simulink library "halout"  (R2021b)
settings: Solver=VariableStepAuto  StartTime=0.0  StopTime=10.0  RelTol=1e-3
undefined symbols (not defined in the file): C_TASK_5MS_S, FALSE, KHAL_CAN1FDAPS3E2E_flg, KHAL_CAN1FDAPS3TxReq_flg, KHAL_CAN1FDVCU2E2E_flg, KHAL_CAN1FDVCU2TxReq_flg, KHAL_CAN1FDVCU3E2E_flg, KHAL_CAN1FDVCU3TxReq_flg, KHAL_CAN1TxReq_flg, KHAL_CAN2TxReq_flg, KHAL_CAN3FDVCU1TxReq_flg, KHAL_CAN3FDVCU2E2E_flg, KHAL_CAN3FDVCU2TxReq_flg, KHAL_CAN3TxReq_flg, KHAL_CAN4FDVCU1E2E_flg, KHAL_CAN4FDVCU1TxReq_flg, KHAL_CAN4TxReq_flg, KHAL_CAN5TxReq_flg, ONE_INT, TRUE, ZERO_INT
libraries: FVT_lib x383, simulink x179
(part 2 of 20)

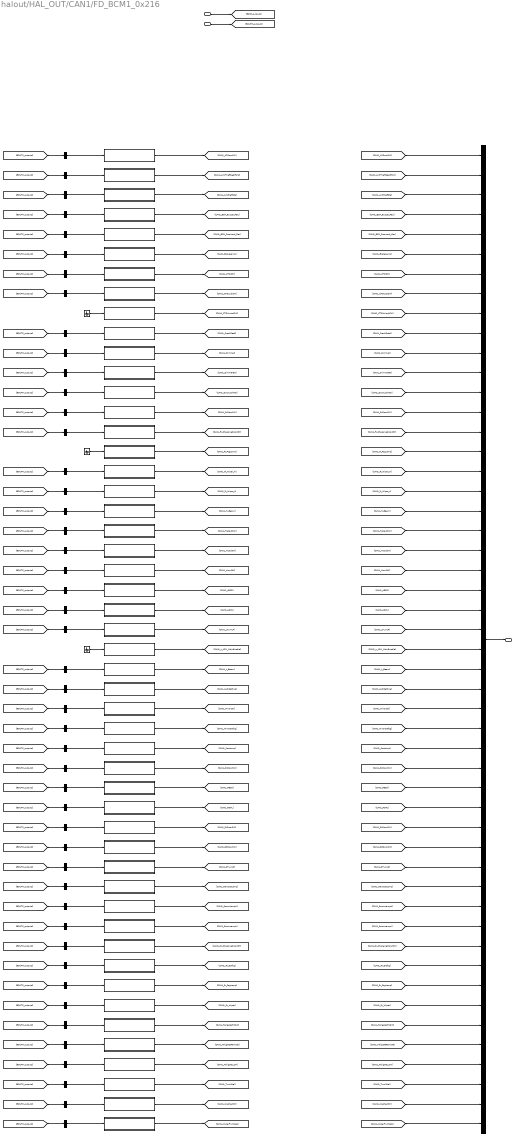
== system halout/HAL_OUT/CAN1/FD_BCM1_0x216 ==
  BSCP_outputs : Inport  OutDataTypeStr=Bus: BSCP_outputs
  BOUTP_outputs : Inport  Port=2  OutDataTypeStr=Bus: BOUTP_outputs
  AllDoorSW : Subsystem
  AntiTheftSeatFold : Subsystem
  AntitheftSta : Subsystem
  BCMBuzzerReq : Subsystem
  BCMDoorLockSta : Subsystem
  BrakeLamp : Subsystem
  CTDCtrl : Subsystem
  CTDLockSW : Subsystem
  CTDUnlockSW : Subsystem
  CrashDetd : Subsystem
  Dimmer : Subsystem
  DimmerEN : Subsystem
  DoorLockIND : Subsystem
  DrDoorSW : Subsystem
  FrChargingDoorCtrl : Subsystem
  FrFogLamp : Subsystem
  FrWiperH : Subsystem
  FrWiperL : Subsystem
  Ground : Ground
  Ground1 : Ground
  Ground2 : Ground
  HBeam : Subsystem
  HazardSW : Subsystem
  HoodSW : Subsystem
  HornCtrl : Subsystem
  LAPMWdwEnable : Subsystem
  LBSD : Subsystem
  LBeam : Subsystem
  LDRL : Subsystem
  LTurnLP : Subsystem
  LockSetting : Subsystem
  MirrorCtrl : Subsystem
  MirrorDefog : Subsystem
  PosLamp : Subsystem
  PsDoorSW : Subsystem
  RBSD : Subsystem
  RDRL : Subsystem
  RLDoorSW : Subsystem
  RRDoorSW : Subsystem
  RTurnLP : Subsystem
  ReverseLamp : Subsystem
  RoomLampH : Subsystem
  RoomLampL : Subsystem
  RrChargingDoorCtrl : Subsystem
  RrDefog : Subsystem
  RrFogLamp : Subsystem
  RrWiper : Subsystem
  TailgateHDSW : Subsystem
  TailgateRemote : Subsystem
  TailgateSW : Subsystem
  TrunkRel : Subsystem
  WasherCtrl : Subsystem
  WiperFixMode : Subsystem
  bus_creator : BusCreator  Inputs=50  OutDataTypeStr=Bus: DT_CAN1_SG_FD_BCM1  NonVirtualBus=on
  bus_selector : BusSelector  OutputSignals=VOUTP_AllDoorSW_flg
  bus_selector1 : BusSelector  OutputSignals=VOUTP_AntitheftSeatFlod_flg
  bus_selector10 : BusSelector  OutputSignals=VOUTP_DimmerEN_flg
  bus_selector11 : BusSelector  OutputSignals=VOUTP_DoorLockIND_flg
  bus_selector12 : BusSelector  OutputSignals=VOUTP_DrDoorSW_flg
  bus_selector13 : BusSelector  OutputSignals=VOUTP_FrChargingDoorCtrl_enum
  bus_selector14 : BusSelector  OutputSignals=VOUTP_FrWiperH_flg
  bus_selector15 : BusSelector  OutputSignals=VOUTP_FrWiperL_flg
  bus_selector16 : BusSelector  OutputSignals=VOUTP_HBeam_flg
  bus_selector17 : BusSelector  OutputSignals=VOUTP_HazardSW_flg
  bus_selector18 : BusSelector  OutputSignals=VOUTP_HoodSW_flg
  bus_selector19 : BusSelector  OutputSignals=VOUTP_HornCtrl_flg
  bus_selector2 : BusSelector  OutputSignals=VOUTP_AntitheftSta_enum
  bus_selector20 : BusSelector  OutputSignals=VOUTP_LBSD_flg
  bus_selector21 : BusSelector  OutputSignals=VOUTP_LDRL_flg
  bus_selector22 : BusSelector  OutputSignals=VOUTP_LTurnLP_flg
  bus_selector23 : BusSelector  OutputSignals=VOUTP_LBeam_flg
  bus_selector24 : BusSelector  OutputSignals=VOUTP_LockSetting_flg
  bus_selector25 : BusSelector  OutputSignals=VOUTP_MirrorCtrl_enum
  bus_selector26 : BusSelector  OutputSignals=VOUTP_MirrorDefog_flg
  bus_selector27 : BusSelector  OutputSignals=VOUTP_PosLamp_flg
  bus_selector28 : BusSelector  OutputSignals=VOUTP_PsDoorSW_flg
  bus_selector29 : BusSelector  OutputSignals=VOUTP_RBSD_flg
  bus_selector3 : BusSelector  OutputSignals=VOUTP_BCMBuzzerReq_flg
  bus_selector30 : BusSelector  OutputSignals=VOUTP_RDRL_flg
  bus_selector31 : BusSelector  OutputSignals=VOUTP_RLDoorSW_flg
  bus_selector32 : BusSelector  OutputSignals=VOUTP_RRDoorSW_flg
  bus_selector33 : BusSelector  OutputSignals=VOUTP_RTurnLP_flg
  bus_selector34 : BusSelector  OutputSignals=VOUTP_ReverseLamp_flg
  bus_selector35 : BusSelector  OutputSignals=VOUTP_RoomLampH_flg
  bus_selector36 : BusSelector  OutputSignals=VOUTP_RoomLampL_flg
  bus_selector37 : BusSelector  OutputSignals=VOUTP_RrChargingDoorCtrl_enum
  bus_selector38 : BusSelector  OutputSignals=VOUTP_RrDefog_flg
  bus_selector39 : BusSelector  OutputSignals=VOUTP_RrFogLamp_flg
  bus_selector4 : BusSelector  OutputSignals=VOUTP_BCMDoorLockSta_flg
  bus_selector40 : BusSelector  OutputSignals=VOUTP_RrWiper_flg
  bus_selector41 : BusSelector  OutputSignals=VOUTP_TailgateHDSW_flg
  bus_selector42 : BusSelector  OutputSignals=VOUTP_TailgateRemote_enum
  bus_selector43 : BusSelector  OutputSignals=VOUTP_TailgateSW_flg
  bus_selector44 : BusSelector  OutputSignals=VOUTP_TrunkRel_flg
  bus_selector45 : BusSelector  OutputSignals=VOUTP_WasherCtrl_enum
  bus_selector46 : BusSelector  OutputSignals=VOUTP_WiperFixMode_flg
  bus_selector5 : BusSelector  OutputSignals=VOUTP_BrakeLamp_flg
  bus_selector6 : BusSelector  OutputSignals=VOUTP_CTDCtrl_enum
  bus_selector7 : BusSelector  OutputSignals=VOUTP_CTDLockSW_flg
  bus_selector8 : BusSelector  OutputSignals=VOUTP_CrashDetd_flg
  bus_selector9 : BusSelector  OutputSignals=VOUTP_Dimmer_pct
  FD_BCM1 : Outport
  wires:
  BSCP_outputs/1 -> [BSCP_outputs]
  BOUTP_outputs/1 -> [BOUTP_outputs]
  [CAN1_AllDoorSW] -> bus_creator/1  "CAN1_AllDoorSW"
  [CAN1_AntiTheftSeatFold] -> bus_creator/2  "CAN1_AntiTheftSeatFold"
  [CAN1_AntitheftSta] -> bus_creator/3  "CAN1_AntitheftSta"
  [CAN1_BCM_Buzzer_Req] -> bus_creator/4  "CAN1_BCM_Buzzer_Req"
  [CAN1_BCM_DoorLock_Sta] -> bus_creator/5  "CAN1_BCM_DoorLock_Sta"
  [CAN1_BrakeLamp] -> bus_creator/6  "CAN1_BrakeLamp"
  [CAN1_CTDCtrl] -> bus_creator/7  "CAN1_CTDCtrl"
  [CAN1_CTDLockSW] -> bus_creator/8  "CAN1_CTDLockSW"
  [CAN1_CTDUnlockSW] -> bus_creator/9  "CAN1_CTDUnlockSW"
  [CAN1_CrashDetd] -> bus_creator/10  "CAN1_CrashDetd"
  [CAN1_Dimmer] -> bus_creator/11  "CAN1_Dimmer"
  [CAN1_DimmerEN] -> bus_creator/12  "CAN1_DimmerEN"
  [CAN1_DoorLockIND] -> bus_creator/13  "CAN1_DoorLockIND"
  [CAN1_DrDoorSW] -> bus_creator/14  "CAN1_DrDoorSW"
  [CAN1_Fr_ChargingDoorCtrl] -> bus_creator/15  "CAN1_Fr_ChargingDoorCtrl"
  [CAN1_Fr_FogLamp] -> bus_creator/16  "CAN1_Fr_FogLamp"
  [CAN1_Fr_Wiper_H] -> bus_creator/17  "CAN1_Fr_Wiper_H"
  [CAN1_Fr_Wiper_L] -> bus_creator/18  "CAN1_Fr_Wiper_L"
  [CAN1_H_Beam] -> bus_creator/19  "CAN1_H_Beam"
  [CAN1_HazardSW] -> bus_creator/20  "CAN1_HazardSW"
  [CAN1_HoodSW] -> bus_creator/21  "CAN1_HoodSW"
  [CAN1_HornCtrl] -> bus_creator/22  "CAN1_HornCtrl"
  [CAN1_LBSD] -> bus_creator/23  "CAN1_LBSD"
  [CAN1_LDRL] -> bus_creator/24  "CAN1_LDRL"
  [CAN1_LTurnLP] -> bus_creator/25  "CAN1_LTurnLP"
  [CAN1_L_APM_WdwEnable] -> bus_creator/26  "CAN1_L_APM_WdwEnable"
  [CAN1_L_Beam] -> bus_creator/27  "CAN1_L_Beam"
  [CAN1_LockSetting] -> bus_creator/28  "CAN1_LockSetting"
  [CAN1_MirrorCtrl] -> bus_creator/29  "CAN1_MirrorCtrl"
  [CAN1_MirrorDefog] -> bus_creator/30  "CAN1_MirrorDefog"
  [CAN1_PosLamp] -> bus_creator/31  "CAN1_PosLamp"
  [CAN1_PsDoorSW] -> bus_creator/32  "CAN1_PsDoorSW"
  [CAN1_RBSD] -> bus_creator/33  "CAN1_RBSD"
  [CAN1_RDRL] -> bus_creator/34  "CAN1_RDRL"
  [CAN1_RLDoorSW] -> bus_creator/35  "CAN1_RLDoorSW"
  [CAN1_RRDoorSW] -> bus_creator/36  "CAN1_RRDoorSW"
  [CAN1_RTurnLP] -> bus_creator/37  "CAN1_RTurnLP"
  [CAN1_ReverseLamp] -> bus_creator/38  "CAN1_ReverseLamp"
  [CAN1_RoomLampH] -> bus_creator/39  "CAN1_RoomLampH"
  [CAN1_RoomLampL] -> bus_creator/40  "CAN1_RoomLampL"
  [CAN1_Rr_ChargingDoorCtrl] -> bus_creator/41  "CAN1_Rr_ChargingDoorCtrl"
  [CAN1_Rr_Defog] -> bus_creator/42  "CAN1_Rr_Defog"
  [CAN1_Rr_FogLamp] -> bus_creator/43  "CAN1_Rr_FogLamp"
  [CAN1_Rr_Wiper] -> bus_creator/44  "CAN1_Rr_Wiper"
  [CAN1_TailgateHDSW] -> bus_creator/45  "CAN1_TailgateHDSW"
  [CAN1_TailgateRemote] -> bus_creator/46  "CAN1_TailgateRemote"
  [CAN1_Tailgate_SW] -> bus_creator/47  "CAN1_Tailgate_SW"
  [CAN1_TrunkRel] -> bus_creator/48  "CAN1_TrunkRel"
  [CAN1_WasherCtrl] -> bus_creator/49  "CAN1_WasherCtrl"
  [CAN1_WiperFixMode] -> bus_creator/50  "CAN1_WiperFixMode"
  bus_creator/1 -> FD_BCM1/1
  AllDoorSW/1(CAN1_AllDoorSW) -> [CAN1_AllDoorSW]
  AntiTheftSeatFold/1(CAN1_AntiTheftSeatFold) -> [CAN1_AntiTheftSeatFold]
  AntitheftSta/1(CAN1_AntitheftSta) -> [CAN1_AntitheftSta]
  BCMBuzzerReq/1(CAN1_BCM_Buzzer_Req) -> [CAN1_BCM_Buzzer_Req]
  BCMDoorLockSta/1(CAN1_BCM_DoorLock_Sta) -> [CAN1_BCM_DoorLock_Sta]
  BrakeLamp/1(CAN1_BrakeLamp) -> [CAN1_BrakeLamp]
  CTDCtrl/1(CAN1_CTDCtrl) -> [CAN1_CTDCtrl]
  CTDLockSW/1(CAN1_CTDLockSW) -> [CAN1_CTDLockSW]
  CTDUnlockSW/1(CAN1_CTDUnlockSW) -> [CAN1_CTDUnlockSW]
  CrashDetd/1(CAN1_CrashDetd) -> [CAN1_CrashDetd]
  Dimmer/1(CAN1_Dimmer) -> [CAN1_Dimmer]
  DimmerEN/1(CAN1_DimmerEN) -> [CAN1_DimmerEN]
  DoorLockIND/1(CAN1_DoorLockIND) -> [CAN1_DoorLockIND]
  DrDoorSW/1(CAN1_DrDoorSW) -> [CAN1_DrDoorSW]
  FrChargingDoorCtrl/1(CAN1_Fr_ChargingDoorCtrl) -> [CAN1_Fr_ChargingDoorCtrl]
  FrFogLamp/1(CAN1_Fr_FogLamp) -> [CAN1_Fr_FogLamp]
  FrWiperH/1(CAN1_Fr_Wiper_H) -> [CAN1_Fr_Wiper_H]
  FrWiperL/1(CAN1_Fr_Wiper_L) -> [CAN1_Fr_Wiper_L]
  HBeam/1(CAN1_H_Beam) -> [CAN1_H_Beam]
  HazardSW/1(CAN1_HazardSW) -> [CAN1_HazardSW]
  HoodSW/1(CAN1_HoodSW) -> [CAN1_HoodSW]
  HornCtrl/1(CAN1_HornCtrl) -> [CAN1_HornCtrl]
  LBSD/1(CAN1_LBSD) -> [CAN1_LBSD]
  LDRL/1(CAN1_LDRL) -> [CAN1_LDRL]
  LTurnLP/1(CAN1_LTurnLP) -> [CAN1_LTurnLP]
  LAPMWdwEnable/1(CAN1_L_APM_WdwEnable) -> [CAN1_L_APM_WdwEnable]
  LBeam/1(CAN1_L_Beam) -> [CAN1_L_Beam]
  LockSetting/1(CAN1_LockSetting) -> [CAN1_LockSetting]
  MirrorCtrl/1(CAN1_MirrorCtrl) -> [CAN1_MirrorCtrl]
  MirrorDefog/1(CAN1_MirrorDefog) -> [CAN1_MirrorDefog]
  PosLamp/1(CAN1_PosLamp) -> [CAN1_PosLamp]
  PsDoorSW/1(CAN1_PsDoorSW) -> [CAN1_PsDoorSW]
  RBSD/1(CAN1_RBSD) -> [CAN1_RBSD]
  RDRL/1(CAN1_RDRL) -> [CAN1_RDRL]
  RLDoorSW/1(CAN1_RLDoorSW) -> [CAN1_RLDoorSW]
  RRDoorSW/1(CAN1_RRDoorSW) -> [CAN1_RRDoorSW]
  RTurnLP/1(CAN1_RTurnLP) -> [CAN1_RTurnLP]
  ReverseLamp/1(CAN1_ReverseLamp) -> [CAN1_ReverseLamp]
  RoomLampH/1(CAN1_RoomLampH) -> [CAN1_RoomLampH]
  RoomLampL/1(CAN1_RoomLampL) -> [CAN1_RoomLampL]
  RrChargingDoorCtrl/1(CAN1_Rr_ChargingDoorCtrl) -> [CAN1_Rr_ChargingDoorCtrl]
  RrDefog/1(CAN1_Rr_Defog) -> [CAN1_Rr_Defog]
  RrFogLamp/1(CAN1_Rr_FogLamp) -> [CAN1_Rr_FogLamp]
  RrWiper/1(CAN1_Rr_Wiper) -> [CAN1_Rr_Wiper]
  TailgateHDSW/1(CAN1_TailgateHDSW) -> [CAN1_TailgateHDSW]
  TailgateRemote/1(CAN1_TailgateRemote) -> [CAN1_TailgateRemote]
  TailgateSW/1(CAN1_Tailgate_SW) -> [CAN1_Tailgate_SW]
  TrunkRel/1(CAN1_TrunkRel) -> [CAN1_TrunkRel]
  WasherCtrl/1(CAN1_WasherCtrl) -> [CAN1_WasherCtrl]
  WiperFixMode/1(CAN1_WiperFixMode) -> [CAN1_WiperFixMode]
  bus_selector/1 -> AllDoorSW/1(AllDoorSW)  "<VOUTP_AllDoorSW_flg>"
  [BOUTP_outputs] -> bus_selector/1
  bus_selector1/1 -> AntiTheftSeatFold/1(AntiTheftSeatFold)  "<VOUTP_AntitheftSeatFlod_flg>"
  [BOUTP_outputs] -> bus_selector1/1
  bus_selector2/1 -> AntitheftSta/1(AntitheftSta)  "<VOUTP_AntitheftSta_enum>"
  [BOUTP_outputs] -> bus_selector2/1
  bus_selector3/1 -> BCMBuzzerReq/1(BCMBuzzerReq)  "<VOUTP_BCMBuzzerReq_flg>"
  [BOUTP_outputs] -> bus_selector3/1
  bus_selector4/1 -> BCMDoorLockSta/1(BCMDoorLockSta)  "<VOUTP_BCMDoorLockSta_flg>"
  [BOUTP_outputs] -> bus_selector4/1
  bus_selector5/1 -> BrakeLamp/1(BrakeLamp)  "<VOUTP_BrakeLamp_flg>"
  [BOUTP_outputs] -> bus_selector5/1
  bus_selector6/1 -> CTDCtrl/1(CTDCtrl)  "<VOUTP_CTDCtrl_enum>"
  [BOUTP_outputs] -> bus_selector6/1
  bus_selector7/1 -> CTDLockSW/1(CTDLockSW)  "<VOUTP_CTDLockSW_flg>"
  [BOUTP_outputs] -> bus_selector7/1
  Ground/1 -> CTDUnlockSW/1(CTDUnlockSW)
  bus_selector8/1 -> CrashDetd/1(CrashDetd)  "<VOUTP_CrashDetd_flg>"
  [BOUTP_outputs] -> bus_selector8/1
  bus_selector9/1 -> Dimmer/1(Dimmer)  "<VOUTP_Dimmer_pct>"
  [BOUTP_outputs] -> bus_selector9/1
  bus_selector10/1 -> DimmerEN/1(DimmerEN)  "<VOUTP_DimmerEN_flg>"
  [BOUTP_outputs] -> bus_selector10/1
  bus_selector11/1 -> DoorLockIND/1(DoorLockIND)  "<VOUTP_DoorLockIND_flg>"
  [BOUTP_outputs] -> bus_selector11/1
  bus_selector12/1 -> DrDoorSW/1(DrDoorSW)  "<VOUTP_DrDoorSW_flg>"
  [BOUTP_outputs] -> bus_selector12/1
  bus_selector13/1 -> FrChargingDoorCtrl/1(FrChargingDoorCtrl)  "<VOUTP_FrChargingDoorCtrl_enum>"
  [BOUTP_outputs] -> bus_selector13/1
  Ground1/1 -> FrFogLamp/1(FrFogLamp)
  bus_selector14/1 -> FrWiperH/1(FrWiperH)  "<VOUTP_FrWiperH_flg>"
  [BOUTP_outputs] -> bus_selector14/1
  bus_selector15/1 -> FrWiperL/1(FrWiperL)  "<VOUTP_FrWiperL_flg>"
  [BOUTP_outputs] -> bus_selector15/1
  bus_selector16/1 -> HBeam/1(HBeam)  "<VOUTP_HBeam_flg>"
  [BOUTP_outputs] -> bus_selector16/1
  bus_selector17/1 -> HazardSW/1(HazardSW)  "<VOUTP_HazardSW_flg>"
  [BOUTP_outputs] -> bus_selector17/1
  bus_selector18/1 -> HoodSW/1(HoodSW)  "<VOUTP_HoodSW_flg>"
  [BOUTP_outputs] -> bus_selector18/1
  bus_selector19/1 -> HornCtrl/1(HornCtrl)  "<VOUTP_HornCtrl_flg>"
  [BOUTP_outputs] -> bus_selector19/1
  bus_selector20/1 -> LBSD/1(LBSD)  "<VOUTP_LBSD_flg>"
  [BOUTP_outputs] -> bus_selector20/1
  bus_selector21/1 -> LDRL/1(LDRL)  "<VOUTP_LDRL_flg>"
  [BOUTP_outputs] -> bus_selector21/1
  bus_selector22/1 -> LTurnLP/1(LTurnLP)  "<VOUTP_LTurnLP_flg>"
  [BOUTP_outputs] -> bus_selector22/1
  Ground2/1 -> LAPMWdwEnable/1(LAPMWdwEnable)
  bus_selector23/1 -> LBeam/1(LBeam)  "<VOUTP_LBeam_flg>"
  [BOUTP_outputs] -> bus_selector23/1
  bus_selector24/1 -> LockSetting/1(LockSetting)  "<VOUTP_LockSetting_flg>"
  [BOUTP_outputs] -> bus_selector24/1
  bus_selector25/1 -> MirrorCtrl/1(MirrorCtrl)  "<VOUTP_MirrorCtrl_enum>"
  [BOUTP_outputs] -> bus_selector25/1
  bus_selector26/1 -> MirrorDefog/1(MirrorDefog)  "<VOUTP_MirrorDefog_flg>"
  [BOUTP_outputs] -> bus_selector26/1
  bus_selector27/1 -> PosLamp/1(PosLamp)  "<VOUTP_PosLamp_flg>"
  [BOUTP_outputs] -> bus_selector27/1
  bus_selector28/1 -> PsDoorSW/1(PsDoorSW)  "<VOUTP_PsDoorSW_flg>"
  [BOUTP_outputs] -> bus_selector28/1
  bus_selector29/1 -> RBSD/1(RBSD)  "<VOUTP_RBSD_flg>"
  [BOUTP_outputs] -> bus_selector29/1
  bus_selector30/1 -> RDRL/1(RDRL)  "<VOUTP_RDRL_flg>"
  [BOUTP_outputs] -> bus_selector30/1
  bus_selector31/1 -> RLDoorSW/1(RLDoorSW)  "<VOUTP_RLDoorSW_flg>"
  [BOUTP_outputs] -> bus_selector31/1
  bus_selector32/1 -> RRDoorSW/1(RRDoorSW)  "<VOUTP_RRDoorSW_flg>"
  [BOUTP_outputs] -> bus_selector32/1
  bus_selector33/1 -> RTurnLP/1(RTurnLP)  "<VOUTP_RTurnLP_flg>"
  [BOUTP_outputs] -> bus_selector33/1
  bus_selector34/1 -> ReverseLamp/1(ReverseLamp)  "<VOUTP_ReverseLamp_flg>"
  [BOUTP_outputs] -> bus_selector34/1
  bus_selector35/1 -> RoomLampH/1(RoomLampH)  "<VOUTP_RoomLampH_flg>"
  [BOUTP_outputs] -> bus_selector35/1
  bus_selector36/1 -> RoomLampL/1(RoomLampL)  "<VOUTP_RoomLampL_flg>"
  [BOUTP_outputs] -> bus_selector36/1
  bus_selector37/1 -> RrChargingDoorCtrl/1(RrChargingDoorCtrl)  "<VOUTP_RrChargingDoorCtrl_enum>"
  [BOUTP_outputs] -> bus_selector37/1
  bus_selector38/1 -> RrDefog/1(RrDefog)  "<VOUTP_RrDefog_flg>"
  [BOUTP_outputs] -> bus_selector38/1
  bus_selector39/1 -> RrFogLamp/1(RrFogLamp)  "<VOUTP_RrFogLamp_flg>"
  [BOUTP_outputs] -> bus_selector39/1
  bus_selector40/1 -> RrWiper/1(RrWiper)  "<VOUTP_RrWiper_flg>"
  [BOUTP_outputs] -> bus_selector40/1
  bus_selector41/1 -> TailgateHDSW/1(TailgateHDSW)  "<VOUTP_TailgateHDSW_flg>"
  [BOUTP_outputs] -> bus_selector41/1
  bus_selector42/1 -> TailgateRemote/1(TailgateRemote)  "<VOUTP_TailgateRemote_enum>"
  [BOUTP_outputs] -> bus_selector42/1
  bus_selector43/1 -> TailgateSW/1(TailgateSW)  "<VOUTP_TailgateSW_flg>"
  [BOUTP_outputs] -> bus_selector43/1
  bus_selector44/1 -> TrunkRel/1(TrunkRel)  "<VOUTP_TrunkRel_flg>"
  [BOUTP_outputs] -> bus_selector44/1
  bus_selector45/1 -> WasherCtrl/1(WasherCtrl)  "<VOUTP_WasherCtrl_enum>"
  [BOUTP_outputs] -> bus_selector45/1
  bus_selector46/1 -> WiperFixMode/1(WiperFixMode)  "<VOUTP_WiperFixMode_flg>"
  [BOUTP_outputs] -> bus_selector46/1

== system halout/HAL_OUT/CAN1/FD_THCM1_0x182 ==
  BSCP_outputs : Inport  OutDataTypeStr=Bus: BSCP_outputs
  BOUTP_outputs : Inport  Port=2  OutDataTypeStr=Bus: BOUTP_outputs
  BatteryMode : Subsystem
  CCUACLampSts : Subsystem
  CCUACMaxLampSts : Subsystem
  CCUAutoLampSts : Subsystem
  CCUAutoMidLampSts : Subsystem
  CCUDispalyRequest : Subsystem
  CCUEcoSts : Subsystem
  CCUFrtOnOffLampSts : Subsystem
  CCUHEATMaxLampSts : Subsystem
  CCURrOnOffLampSts : Subsystem
  CCUSyncLampSts : Subsystem
  CabinMode : Subsystem
  EDriveMode : Subsystem
  FDAGSCmd : Subsystem
  FDRecyAutoCmd : Subsystem
  FrCoolantflow : Subsystem
  FrCoolanttemp : Subsystem
  Ground{,1..17} (18 alike) : Ground
  HPThermalRecoveryReq : Subsystem
  RrCoolantflow : Subsystem
  RrCoolanttemp : Subsystem
  bus_creator : BusCreator  Inputs=37  OutDataTypeStr=Bus: DT_CAN1_SG_FD_THCM1  NonVirtualBus=on
  bus_selector : BusSelector  OutputSignals=VOUTP_BatteryMode_enum
  bus_selector1 : BusSelector  OutputSignals=VOUTP_CCUACLampSts_flg
  bus_selector10 : BusSelector  OutputSignals=VOUTP_sigAmbAirT_C
  bus_selector11 : BusSelector  OutputSignals=VOUTP_sigCbnAirT_C
  bus_selector12 : BusSelector  OutputSignals=VOUTP_sigCbnSolarLeft_W
  bus_selector13 : BusSelector  OutputSignals=VOUTP_sigCbnSolarRight_W
  bus_selector14 : BusSelector  OutputSignals=VOUTP_sigClntTHvBattOut_C
  bus_selector15 : BusSelector  OutputSignals=VOUTP_sigRecircSt_flg
  bus_selector16 : BusSelector  OutputSignals=VOUTP_sigSetTempZon1St_C
  bus_selector17 : BusSelector  OutputSignals=VOUTP_sigSetTempZon2St_C
  bus_selector18 : BusSelector  OutputSignals=VOUTP_sigWindDirZon1St_enum
  bus_selector2 : BusSelector  OutputSignals=VOUTP_CCUACMaxLampSts_flg
  bus_selector3 : BusSelector  OutputSignals=VOUTP_CCUAutoLampSts_flg
  bus_selector4 : BusSelector  OutputSignals=VOUTP_CCUSyncLampSts_flg
  bus_selector5 : BusSelector  OutputSignals=VOUTP_CabinMode_enum
  bus_selector6 : BusSelector  OutputSignals=VOUTP_EDriveMode_enum
  bus_selector7 : BusSelector  OutputSignals=VOUTP_FDAGSCmd_enum
  bus_selector8 : BusSelector  OutputSignals=VOUTP_FDRecyAutoCmd_enum
  bus_selector9 : BusSelector  OutputSignals=VOUTP_sigAirIntenZon1St_enum
  sigAirIntenZon1St : Subsystem
  sigAirIntenZon3St : Subsystem
  sigAmbAirT : Subsystem
  sigCbnAirT : Subsystem
  sigCbnPTCPwrAct : Subsystem
  sigCbnSolarLeft : Subsystem
  sigCbnSolarRight : Subsystem
  sigClmtCmprPwrAct : Subsystem
  sigClntTHvBattOut : Subsystem
  sigDfrstSt : Subsystem
  sigHvacSt : Subsystem
  sigRecircSt : Subsystem
  sigSetTempZon1St : Subsystem
  sigSetTempZon2St : Subsystem
  sigSetTempZon3St : Subsystem
  sigWindDirZon1St : Subsystem
  sigWindDirZon3St : Subsystem
  FD_THCM1 : Outport
  wires:
  BSCP_outputs/1 -> [BSCP_outputs]
  BOUTP_outputs/1 -> [BOUTP_outputs]
  [CAN1_BatteryMode] -> bus_creator/1  "CAN1_BatteryMode"
  [CAN1_CCU_ACLampSts] -> bus_creator/2  "CAN1_CCU_ACLampSts"
  [CAN1_CCU_ACMaxLampSts] -> bus_creator/3  "CAN1_CCU_ACMaxLampSts"
  [CAN1_CCU_AutoLampSts] -> bus_creator/4  "CAN1_CCU_AutoLampSts"
  [CAN1_CCU_AutoMidLampSts] -> bus_creator/5  "CAN1_CCU_AutoMidLampSts"
  [CAN1_CCU_Dispaly_Request] -> bus_creator/6  "CAN1_CCU_Dispaly_Request"
  [CAN1_CCU_EcoSts] -> bus_creator/7  "CAN1_CCU_EcoSts"
  [CAN1_CCU_FrtOnOffLampSts] -> bus_creator/8  "CAN1_CCU_FrtOnOffLampSts"
  [CAN1_CCU_HEATMaxLampSts] -> bus_creator/9  "CAN1_CCU_HEATMaxLampSts"
  [CAN1_CCU_RrOnOffLampSts] -> bus_creator/10  "CAN1_CCU_RrOnOffLampSts"
  [CAN1_CCU_SyncLampSts] -> bus_creator/11  "CAN1_CCU_SyncLampSts"
  [CAN1_CabinMode] -> bus_creator/12  "CAN1_CabinMode"
  [CAN1_EDriveMode] -> bus_creator/13  "CAN1_EDriveMode"
  [CAN1_FD_AGS_Cmd] -> bus_creator/14  "CAN1_FD_AGS_Cmd"
  [CAN1_FD_RecyAuto_Cmd] -> bus_creator/15  "CAN1_FD_RecyAuto_Cmd"
  [CAN1_Fr_Coolantflow] -> bus_creator/16  "CAN1_Fr_Coolantflow"
  [CAN1_Fr_Coolanttemp] -> bus_creator/17  "CAN1_Fr_Coolanttemp"
  [CAN1_HPThermalRecoveryReq] -> bus_creator/18  "CAN1_HPThermalRecoveryReq"
  [CAN1_Rr_Coolantflow] -> bus_creator/19  "CAN1_Rr_Coolantflow"
  [CAN1_Rr_Coolanttemp] -> bus_creator/20  "CAN1_Rr_Coolanttemp"
  [CAN1_sigAirIntenZon1St] -> bus_creator/21  "CAN1_sigAirIntenZon1St"
  [CAN1_sigAirIntenZon3St] -> bus_creator/22  "CAN1_sigAirIntenZon3St"
  [CAN1_sigAmbAirT] -> bus_creator/23  "CAN1_sigAmbAirT"
  [CAN1_sigCbnAirT] -> bus_creator/24  "CAN1_sigCbnAirT"
  [CAN1_sigCbnPTCPwrAct] -> bus_creator/25  "CAN1_sigCbnPTCPwrAct"
  [CAN1_sigCbnSolarLeft] -> bus_creator/26  "CAN1_sigCbnSolarLeft"
  [CAN1_sigCbnSolarRight] -> bus_creator/27  "CAN1_sigCbnSolarRight"
  [CAN1_sigClmtCmprPwrAct] -> bus_creator/28  "CAN1_sigClmtCmprPwrAct"
  [CAN1_sigClntTHvBattOut] -> bus_creator/29  "CAN1_sigClntTHvBattOut"
  [CAN1_sigDfrstSt] -> bus_creator/30  "CAN1_sigDfrstSt"
  [CAN1_sigHvacSt] -> bus_creator/31  "CAN1_sigHvacSt"
  [CAN1_sigRecircSt] -> bus_creator/32  "CAN1_sigRecircSt"
  [CAN1_sigSetTempZon1St] -> bus_creator/33  "CAN1_sigSetTempZon1St"
  [CAN1_sigSetTempZon2St] -> bus_creator/34  "CAN1_sigSetTempZon2St"
  [CAN1_sigSetTempZon3St] -> bus_creator/35  "CAN1_sigSetTempZon3St"
  [CAN1_sigWindDirZon1St] -> bus_creator/36  "CAN1_sigWindDirZon1St"
  [CAN1_sigWindDirZon3St] -> bus_creator/37  "CAN1_sigWindDirZon3St"
  bus_creator/1 -> FD_THCM1/1
  BatteryMode/1(CAN1_BatteryMode) -> [CAN1_BatteryMode]
  CCUACLampSts/1(CAN1_CCU_ACLampSts) -> [CAN1_CCU_ACLampSts]
  CCUACMaxLampSts/1(CAN1_CCU_ACMaxLampSts) -> [CAN1_CCU_ACMaxLampSts]
  CCUAutoLampSts/1(CAN1_CCU_AutoLampSts) -> [CAN1_CCU_AutoLampSts]
  CCUAutoMidLampSts/1(CAN1_CCU_AutoMidLampSts) -> [CAN1_CCU_AutoMidLampSts]
  CCUDispalyRequest/1(CAN1_CCU_Dispaly_Request) -> [CAN1_CCU_Dispaly_Request]
  CCUEcoSts/1(CAN1_CCU_EcoSts) -> [CAN1_CCU_EcoSts]
  CCUFrtOnOffLampSts/1(CAN1_CCU_FrtOnOffLampSts) -> [CAN1_CCU_FrtOnOffLampSts]
  CCUHEATMaxLampSts/1(CAN1_CCU_HEATMaxLampSts) -> [CAN1_CCU_HEATMaxLampSts]
  CCURrOnOffLampSts/1(CAN1_CCU_RrOnOffLampSts) -> [CAN1_CCU_RrOnOffLampSts]
  CCUSyncLampSts/1(CAN1_CCU_SyncLampSts) -> [CAN1_CCU_SyncLampSts]
  CabinMode/1(CAN1_CabinMode) -> [CAN1_CabinMode]
  EDriveMode/1(CAN1_EDriveMode) -> [CAN1_EDriveMode]
  FDAGSCmd/1(CAN1_FD_AGS_Cmd) -> [CAN1_FD_AGS_Cmd]
  FDRecyAutoCmd/1(CAN1_FD_RecyAuto_Cmd) -> [CAN1_FD_RecyAuto_Cmd]
  FrCoolantflow/1(CAN1_Fr_Coolantflow) -> [CAN1_Fr_Coolantflow]
  FrCoolanttemp/1(CAN1_Fr_Coolanttemp) -> [CAN1_Fr_Coolanttemp]
  HPThermalRecoveryReq/1(CAN1_HPThermalRecoveryReq) -> [CAN1_HPThermalRecoveryReq]
  RrCoolantflow/1(CAN1_Rr_Coolantflow) -> [CAN1_Rr_Coolantflow]
  RrCoolanttemp/1(CAN1_Rr_Coolanttemp) -> [CAN1_Rr_Coolanttemp]
  sigAirIntenZon1St/1(CAN1_sigAirIntenZon1St) -> [CAN1_sigAirIntenZon1St]
  sigAirIntenZon3St/1(CAN1_sigAirIntenZon3St) -> [CAN1_sigAirIntenZon3St]
  sigAmbAirT/1(CAN1_sigAmbAirT) -> [CAN1_sigAmbAirT]
  sigCbnAirT/1(CAN1_sigCbnAirT) -> [CAN1_sigCbnAirT]
  sigCbnPTCPwrAct/1(CAN1_sigCbnPTCPwrAct) -> [CAN1_sigCbnPTCPwrAct]
  sigCbnSolarLeft/1(CAN1_sigCbnSolarLeft) -> [CAN1_sigCbnSolarLeft]
  sigCbnSolarRight/1(CAN1_sigCbnSolarRight) -> [CAN1_sigCbnSolarRight]
  sigClmtCmprPwrAct/1(CAN1_sigClmtCmprPwrAct) -> [CAN1_sigClmtCmprPwrAct]
  sigClntTHvBattOut/1(CAN1_sigClntTHvBattOut) -> [CAN1_sigClntTHvBattOut]
  sigDfrstSt/1(CAN1_sigDfrstSt) -> [CAN1_sigDfrstSt]
  sigHvacSt/1(CAN1_sigHvacSt) -> [CAN1_sigHvacSt]
  sigRecircSt/1(CAN1_sigRecircSt) -> [CAN1_sigRecircSt]
  sigSetTempZon1St/1(CAN1_sigSetTempZon1St) -> [CAN1_sigSetTempZon1St]
  sigSetTempZon2St/1(CAN1_sigSetTempZon2St) -> [CAN1_sigSetTempZon2St]
  sigSetTempZon3St/1(CAN1_sigSetTempZon3St) -> [CAN1_sigSetTempZon3St]
  sigWindDirZon1St/1(CAN1_sigWindDirZon1St) -> [CAN1_sigWindDirZon1St]
  sigWindDirZon3St/1(CAN1_sigWindDirZon3St) -> [CAN1_sigWindDirZon3St]
  bus_selector/1 -> BatteryMode/1(BatteryMode)  "<VOUTP_BatteryMode_enum>"
  [BOUTP_outputs] -> bus_selector/1
  bus_selector1/1 -> CCUACLampSts/1(CCUACLampSts)  "<VOUTP_CCUACLampSts_flg>"
  [BOUTP_outputs] -> bus_selector1/1
  bus_selector2/1 -> CCUACMaxLampSts/1(CCUACMaxLampSts)  "<VOUTP_CCUACMaxLampSts_flg>"
  [BOUTP_outputs] -> bus_selector2/1
  bus_selector3/1 -> CCUAutoLampSts/1(CCUAutoLampSts)  "<VOUTP_CCUAutoLampSts_flg>"
  [BOUTP_outputs] -> bus_selector3/1
  Ground/1 -> CCUAutoMidLampSts/1(CCUAutoMidLampSts)
  Ground1/1 -> CCUDispalyRequest/1(CCUDispalyRequest)
  Ground2/1 -> CCUEcoSts/1(CCUEcoSts)
  Ground3/1 -> CCUFrtOnOffLampSts/1(CCUFrtOnOffLampSts)
  Ground4/1 -> CCUHEATMaxLampSts/1(CCUHEATMaxLampSts)
  Ground5/1 -> CCURrOnOffLampSts/1(CCURrOnOffLampSts)
  bus_selector4/1 -> CCUSyncLampSts/1(CCUSyncLampSts)  "<VOUTP_CCUSyncLampSts_flg>"
  [BOUTP_outputs] -> bus_selector4/1
  bus_selector5/1 -> CabinMode/1(CabinMode)  "<VOUTP_CabinMode_enum>"
  [BOUTP_outputs] -> bus_selector5/1
  bus_selector6/1 -> EDriveMode/1(EDriveMode)  "<VOUTP_EDriveMode_enum>"
  [BOUTP_outputs] -> bus_selector6/1
  bus_selector7/1 -> FDAGSCmd/1(FDAGSCmd)  "<VOUTP_FDAGSCmd_enum>"
  [BOUTP_outputs] -> bus_selector7/1
  bus_selector8/1 -> FDRecyAutoCmd/1(FDRecyAutoCmd)  "<VOUTP_FDRecyAutoCmd_enum>"
  [BOUTP_outputs] -> bus_selector8/1
  Ground6/1 -> FrCoolantflow/1(FrCoolantflow)
  Ground7/1 -> FrCoolanttemp/1(FrCoolanttemp)
  Ground8/1 -> HPThermalRecoveryReq/1(HPThermalRecoveryReq)
  Ground9/1 -> RrCoolantflow/1(RrCoolantflow)
  Ground10/1 -> RrCoolanttemp/1(RrCoolanttemp)
  bus_selector9/1 -> sigAirIntenZon1St/1(sigAirIntenZon1St)  "<VOUTP_sigAirIntenZon1St_enum>"
  [BOUTP_outputs] -> bus_selector9/1
  Ground11/1 -> sigAirIntenZon3St/1(sigAirIntenZon3St)
  bus_selector10/1 -> sigAmbAirT/1(sigAmbAirT)  "<VOUTP_sigAmbAirT_C>"
  [BOUTP_outputs] -> bus_selector10/1
  bus_selector11/1 -> sigCbnAirT/1(sigCbnAirT)  "<VOUTP_sigCbnAirT_C>"
  [BOUTP_outputs] -> bus_selector11/1
  Ground12/1 -> sigCbnPTCPwrAct/1(sigCbnPTCPwrAct)
  bus_selector12/1 -> sigCbnSolarLeft/1(sigCbnSolarLeft)  "<VOUTP_sigCbnSolarLeft_W>"
  [BOUTP_outputs] -> bus_selector12/1
  bus_selector13/1 -> sigCbnSolarRight/1(sigCbnSolarRight)  "<VOUTP_sigCbnSolarRight_W>"
  [BOUTP_outputs] -> bus_selector13/1
  Ground13/1 -> sigClmtCmprPwrAct/1(sigClmtCmprPwrAct)
  bus_selector14/1 -> sigClntTHvBattOut/1(sigClntTHvBattOut)  "<VOUTP_sigClntTHvBattOut_C>"
  [BOUTP_outputs] -> bus_selector14/1
  Ground14/1 -> sigDfrstSt/1(sigDfrstSt)
  Ground15/1 -> sigHvacSt/1(sigHvacSt)
  bus_selector15/1 -> sigRecircSt/1(sigRecircSt)  "<VOUTP_sigRecircSt_flg>"
  [BOUTP_outputs] -> bus_selector15/1
  bus_selector16/1 -> sigSetTempZon1St/1(sigSetTempZon1St)  "<VOUTP_sigSetTempZon1St_C>"
  [BOUTP_outputs] -> bus_selector16/1
  bus_selector17/1 -> sigSetTempZon2St/1(sigSetTempZon2St)  "<VOUTP_sigSetTempZon2St_C>"
  [BOUTP_outputs] -> bus_selector17/1
  Ground16/1 -> sigSetTempZon3St/1(sigSetTempZon3St)
  bus_selector18/1 -> sigWindDirZon1St/1(sigWindDirZon1St)  "<VOUTP_sigWindDirZon1St_enum>"
  [BOUTP_outputs] -> bus_selector18/1
  Ground17/1 -> sigWindDirZon3St/1(sigWindDirZon3St)

== system halout/HAL_OUT/CAN1/FD_VCU1_0x116 ==
  BSCP_outputs : Inport  OutDataTypeStr=Bus: BSCP_outputs
  BOUTP_outputs : Inport  Port=2  OutDataTypeStr=Bus: BOUTP_outputs
  CCCrlSta : Subsystem
  Ground : Ground
  HVPwrSta : Subsystem
  LVPwrSta : Subsystem
  MSACrlSta : Subsystem
  PButtonSta : Subsystem
  PrkReq : Subsystem
  PrkReqValid : Subsystem
  PwrSta : Subsystem
  ShiftGearPosn : Subsystem
  XWDMode : Subsystem
  bus_creator : BusCreator  Inputs=10  OutDataTypeStr=Bus: DT_CAN1_SG_FD_VCU1  NonVirtualBus=on
  bus_selector : BusSelector  OutputSignals=VOUTP_CCCtrlSta_enum
  bus_selector1 : BusSelector  OutputSignals=VOUTP_HVPwrSta_flg
  bus_selector2 : BusSelector  OutputSignals=VOUTP_LVPwrSta_flg
  bus_selector3 : BusSelector  OutputSignals=VOUTP_MSACtrlSta_enum
  bus_selector4 : BusSelector  OutputSignals=VOUTP_PButtonSta_enum
  bus_selector5 : BusSelector  OutputSignals=VOUTP_ActParkRequest_flg
  bus_selector6 : BusSelector  OutputSignals=VOUTP_PowerSta_enum
  bus_selector7 : BusSelector  OutputSignals=VOUTP_ShiftGearPosn_enum
  bus_selector8 : BusSelector  OutputSignals=VOUTP_DrivetrainSelect_enum
  FD_VCU1 : Outport
  wires:
  BSCP_outputs/1 -> [BSCP_outputs]
  BOUTP_outputs/1 -> [BOUTP_outputs]
  [CAN1_CC_Crl_Sta] -> bus_creator/1  "CAN1_CC_Crl_Sta"
  [CAN1_HVPwrSta] -> bus_creator/2  "CAN1_HVPwrSta"
  [CAN1_LVPwrSta] -> bus_creator/3  "CAN1_LVPwrSta"
  [CAN1_MSA_Crl_Sta] -> bus_creator/4  "CAN1_MSA_Crl_Sta"
  [CAN1_P_Button_Sta] -> bus_creator/5  "CAN1_P_Button_Sta"
  [CAN1_PrkReq] -> bus_creator/6  "CAN1_PrkReq"
  [CAN1_PrkReqValid] -> bus_creator/7  "CAN1_PrkReqValid"
  [CAN1_PwrSta] -> bus_creator/8  "CAN1_PwrSta"
  [CAN1_ShiftGearPosn] -> bus_creator/9  "CAN1_ShiftGearPosn"
  [CAN1_XWDMode] -> bus_creator/10  "CAN1_XWDMode"
  bus_creator/1 -> FD_VCU1/1
  CCCrlSta/1(CAN1_CC_Crl_Sta) -> [CAN1_CC_Crl_Sta]
  HVPwrSta/1(CAN1_HVPwrSta) -> [CAN1_HVPwrSta]
  LVPwrSta/1(CAN1_LVPwrSta) -> [CAN1_LVPwrSta]
  MSACrlSta/1(CAN1_MSA_Crl_Sta) -> [CAN1_MSA_Crl_Sta]
  PButtonSta/1(CAN1_P_Button_Sta) -> [CAN1_P_Button_Sta]
  PrkReq/1(CAN1_PrkReq) -> [CAN1_PrkReq]
  PrkReqValid/1(CAN1_PrkReqValid) -> [CAN1_PrkReqValid]
  PwrSta/1(CAN1_PwrSta) -> [CAN1_PwrSta]
  ShiftGearPosn/1(CAN1_ShiftGearPosn) -> [CAN1_ShiftGearPosn]
  XWDMode/1(CAN1_XWDMode) -> [CAN1_XWDMode]
  bus_selector/1 -> CCCrlSta/1(CCCrlSta)  "<VOUTP_CCCtrlSta_enum>"
  [BOUTP_outputs] -> bus_selector/1
  bus_selector1/1 -> HVPwrSta/1(HVPwrSta)  "<VOUTP_HVPwrSta_flg>"
  [BOUTP_outputs] -> bus_selector1/1
  bus_selector2/1 -> LVPwrSta/1(LVPwrSta)  "<VOUTP_LVPwrSta_flg>"
  [BOUTP_outputs] -> bus_selector2/1
  bus_selector3/1 -> MSACrlSta/1(MSACrlSta)  "<VOUTP_MSACtrlSta_enum>"
  [BOUTP_outputs] -> bus_selector3/1
  bus_selector4/1 -> PButtonSta/1(PButtonSta)  "<VOUTP_PButtonSta_enum>"
  [BOUTP_outputs] -> bus_selector4/1
  bus_selector5/1 -> PrkReq/1(PrkReq)  "<VOUTP_ActParkRequest_flg>"
  [BOUTP_outputs] -> bus_selector5/1
  Ground/1 -> PrkReqValid/1(PrkReqValid)
  bus_selector6/1 -> PwrSta/1(PwrSta)  "<VOUTP_PowerSta_enum>"
  [BOUTP_outputs] -> bus_selector6/1
  bus_selector7/1 -> ShiftGearPosn/1(ShiftGearPosn)  "<VOUTP_ShiftGearPosn_enum>"
  [BOUTP_outputs] -> bus_selector7/1
  bus_selector8/1 -> XWDMode/1(XWDMode)  "<VOUTP_DrivetrainSelect_enum>"
  [BOUTP_outputs] -> bus_selector8/1

== system halout/HAL_OUT/CAN1/FD_VCU2_0x154 ==
  BSCP_outputs : Inport  OutDataTypeStr=Bus: BSCP_outputs
  BOUTP_outputs : Inport  Port=2  OutDataTypeStr=Bus: BOUTP_outputs
  Trigger : TriggerPort  TriggerType=function-call  VariantControl=(inherit)
  ACCCtrlAvail : Subsystem
  AccPedalOverride : Subsystem
  ActAPSPosn : Subsystem
  Byte_0 : Subsystem
  Byte_1 : Subsystem
  Byte_10 : Subsystem
  Byte_11 : Subsystem
  Byte_12 : Subsystem
  Byte_13 : Subsystem
  Byte_14 : Subsystem
  Byte_15 : Subsystem
  Byte_2 : Subsystem
  Byte_3 : Subsystem
  Byte_4 : Subsystem
  Byte_5 : Subsystem
  Byte_{6..9} (4 alike) : Constant  Value=ZERO_INT
  CRC8_IfAction_Tx : FVT_lib/hal/CRC8_IfAction_Tx
  CSVCU2CAN1 : Subsystem
  Constant : Constant  Value=KHAL_CAN1FDVCU2E2E_flg
  Constant1 : Constant  Value=0xf1
  Constant2 : Constant  Value=0xf8
  Constant3 : Constant  Value=KHAL_CAN1FDVCU2E2E_flg
  Constant4 : Constant  Value=KHAL_CAN1FDVCU2E2E_flg
  DriverTq : Subsystem
  FrDriverTq : Subsystem
  Ground{,1..7} (8 alike) : Ground
  Mux2 : Mux  Inputs=15
  RCVCU2CAN1 : Subsystem
  RollingCounter_IfAction : FVT_lib/hal/RollingCounter_IfAction
  RollingCounter_IfAction1 : FVT_lib/hal/RollingCounter_IfAction
  RrDriverTq : Subsystem
  Terminator : Terminator
  VehActPwr : Subsystem
  bus_creator : BusCreator  Inputs=9  OutDataTypeStr=Bus: DT_CAN1_SG_FD_VCU2  NonVirtualBus=on
  bus_selector : BusSelector  OutputSignals=VOUTP_ACCCtrlAvail_flg
  bus_selector1 : BusSelector  OutputSignals=VOUTP_ACCPedalOvrd_flg
  bus_selector10 : BusSelector  OutputSignals=VOUTP_DriverWhlTqDemFr_Nm
  bus_selector11 : BusSelector  OutputSignals=VOUTP_DriverWhlTqDemRr_Nm
  bus_selector2 : BusSelector  OutputSignals=VOUTP_DriverWhlTqDemFr_Nm
  bus_selector3 : BusSelector  OutputSignals=VOUTP_DriverWhlTqDemFr_Nm
  bus_selector4 : BusSelector  OutputSignals=VOUTP_DriverWhlTqDemRr_Nm
  bus_selector5 : BusSelector  OutputSignals=VOUTP_DriverWhlTqDemRr_Nm
  bus_selector6 : BusSelector  OutputSignals=VOUTP_ActAPSPosn_pct
  bus_selector7 : BusSelector  OutputSignals=VOUTP_ACCCtrlAvail_flg
  bus_selector8 : BusSelector  OutputSignals=VOUTP_ACCPedalOvrd_flg
  bus_selector9 : BusSelector  OutputSignals=VOUTP_ActAPSPosn_pct
  FD_VCU2 : Outport
  wires:
  BSCP_outputs/1 -> [BSCP_outputs]
  BOUTP_outputs/1 -> [BOUTP_outputs]
  [CAN1_ACC_CtrlAvail] -> bus_creator/1  "CAN1_ACC_CtrlAvail"
  [CAN1_AccPedal_Override] -> bus_creator/2  "CAN1_AccPedal_Override"
  [CAN1_ActAPSPosn] -> bus_creator/3  "CAN1_ActAPSPosn"
  [CAN1_CS_VCU2_CAN1] -> bus_creator/4  "CAN1_CS_VCU2_CAN1"
  [CAN1_DriverTq] -> bus_creator/5  "CAN1_DriverTq"
  [CAN1_Fr_DriverTq] -> bus_creator/6  "CAN1_Fr_DriverTq"
  [CAN1_RC_VCU2_CAN1] -> bus_creator/7  "CAN1_RC_VCU2_CAN1"
  [CAN1_Rr_DriverTq] -> bus_creator/8  "CAN1_Rr_DriverTq"
  [CAN1_VehActPwr] -> bus_creator/9  "CAN1_VehActPwr"
  bus_creator/1 -> FD_VCU2/1
  ACCCtrlAvail/1(CAN1_ACC_CtrlAvail) -> [CAN1_ACC_CtrlAvail]
  AccPedalOverride/1(CAN1_AccPedal_Override) -> [CAN1_AccPedal_Override]
  ActAPSPosn/1(CAN1_ActAPSPosn) -> [CAN1_ActAPSPosn]
  CSVCU2CAN1/1(CAN1_CS_VCU2_CAN1) -> [CAN1_CS_VCU2_CAN1]
  DriverTq/1(CAN1_DriverTq) -> [CAN1_DriverTq]
  FrDriverTq/1(CAN1_Fr_DriverTq) -> [CAN1_Fr_DriverTq]
  RCVCU2CAN1/1(CAN1_RC_VCU2_CAN1) -> [CAN1_RC_VCU2_CAN1]
  RrDriverTq/1(CAN1_Rr_DriverTq) -> [CAN1_Rr_DriverTq]
  VehActPwr/1(CAN1_VehActPwr) -> [CAN1_VehActPwr]
  Byte_0/1(Byte_0) -> Terminator/1
  Byte_1/1(Byte_1) -> [Byte_1]
  Byte_2/1(Byte_2) -> [Byte_2]
  Byte_3/1(Byte_3) -> [Byte_3]
  Byte_4/1(Byte_4) -> [Byte_4]
  Byte_5/1(Byte_5) -> [Byte_5]
  Byte_6/1 -> [Byte_6]
  Byte_7/1 -> [Byte_7]
  Byte_8/1 -> [Byte_8]
  Byte_9/1 -> [Byte_9]
  Byte_10/1(Byte_10) -> [Byte_10]
  Byte_11/1(Byte_11) -> [Byte_11]
  Byte_12/1(Byte_12) -> [Byte_12]
  Byte_13/1(Byte_13) -> [Byte_13]
  Byte_14/1(Byte_14) -> [Byte_14]
  Byte_15/1(Byte_15) -> [Byte_15]
  Mux2/1 -> CRC8_IfAction_Tx/4
  Constant/1 -> CRC8_IfAction_Tx/1
  Constant1/1 -> CRC8_IfAction_Tx/2
  Constant2/1 -> CRC8_IfAction_Tx/3
  CRC8_IfAction_Tx/1 -> [CS_VCU2_CAN1]
  Ground/1 -> Byte_0/1(CS_VCU2_CAN1)
  [Byte_1] -> Mux2/1
  bus_selector/1 -> Byte_1/1(ACC_CtrlAvail)  "<VOUTP_ACCCtrlAvail_flg>"
  [BOUTP_outputs] -> bus_selector/1
  bus_selector1/1 -> Byte_1/2(AccPedal_Override)  "<VOUTP_ACCPedalOvrd_flg>"
  [BOUTP_outputs] -> bus_selector1/1
  RollingCounter_IfAction/1 -> Byte_1/3(RC_VCU2_CAN1)
  Constant3/1 -> RollingCounter_IfAction/1
  [Byte_2] -> Mux2/2
  bus_selector2/1 -> Byte_2/1(Fr_DriverTq)  "<VOUTP_DriverWhlTqDemFr_Nm>"
  [BOUTP_outputs] -> bus_selector2/1
  [Byte_3] -> Mux2/3
  bus_selector3/1 -> Byte_3/1(Fr_DriverTq)  "<VOUTP_DriverWhlTqDemFr_Nm>"
  [BOUTP_outputs] -> bus_selector3/1
  [Byte_4] -> Mux2/4
  bus_selector4/1 -> Byte_4/1(Rr_DriverTq)  "<VOUTP_DriverWhlTqDemRr_Nm>"
  [BOUTP_outputs] -> bus_selector4/1
  [Byte_5] -> Mux2/5
  bus_selector5/1 -> Byte_5/1(Rr_DriverTq)  "<VOUTP_DriverWhlTqDemRr_Nm>"
  [BOUTP_outputs] -> bus_selector5/1
  [Byte_6] -> Mux2/6
  [Byte_7] -> Mux2/7
  [Byte_8] -> Mux2/8
  [Byte_9] -> Mux2/9
  [Byte_10] -> Mux2/10
  Ground1/1 -> Byte_10/1(VehActPwr)
  [Byte_11] -> Mux2/11
  Ground2/1 -> Byte_11/1(VehActPwr)
  [Byte_12] -> Mux2/12
  Ground3/1 -> Byte_12/1(VehActPwr)
  [Byte_13] -> Mux2/13
  Ground4/1 -> Byte_13/1(DriverTq)
  [Byte_14] -> Mux2/14
  Ground5/1 -> Byte_14/1(DriverTq)
  [Byte_15] -> Mux2/15
  bus_selector6/1 -> Byte_15/1(ActAPSPosn)  "<VOUTP_ActAPSPosn_pct>"
  [BOUTP_outputs] -> bus_selector6/1
  bus_selector7/1 -> ACCCtrlAvail/1(ACCCtrlAvail)  "<VOUTP_ACCCtrlAvail_flg>"
  [BOUTP_outputs] -> bus_selector7/1
  bus_selector8/1 -> AccPedalOverride/1(AccPedalOverride)  "<VOUTP_ACCPedalOvrd_flg>"
  [BOUTP_outputs] -> bus_selector8/1
  bus_selector9/1 -> ActAPSPosn/1(ActAPSPosn)  "<VOUTP_ActAPSPosn_pct>"
  [BOUTP_outputs] -> bus_selector9/1
  [CS_VCU2_CAN1] -> CSVCU2CAN1/1(CSVCU2CAN1)
  Ground6/1 -> DriverTq/1(DriverTq)
  bus_selector10/1 -> FrDriverTq/1(FrDriverTq)  "<VOUTP_DriverWhlTqDemFr_Nm>"
  [BOUTP_outputs] -> bus_selector10/1
  RollingCounter_IfAction1/1 -> RCVCU2CAN1/1(RCVCU2CAN1)
  Constant4/1 -> RollingCounter_IfAction1/1
  bus_selector11/1 -> RrDriverTq/1(RrDriverTq)  "<VOUTP_DriverWhlTqDemRr_Nm>"
  [BOUTP_outputs] -> bus_selector11/1
  Ground7/1 -> VehActPwr/1(VehActPwr)

== system halout/HAL_OUT/CAN1/FD_VCU2_Tx ==
  TxReq : Inport
  Chart : Stateflow chart  TreatAsAtomicUnit=on
  Constant : Constant  Value=C_TASK_5MS_S
  Constant3 : Constant  Value=CycleTime
  Data Type Conversion : DataTypeConversion  OutDataTypeStr=uint16
  Divide : Product  Inputs=*/
  Gain : Gain  Gain=0.001
  TxTrigger : Outport
  wires:
  Data Type Conversion/1 -> Chart/2(CycleCnt)
  Constant3/1 -> Gain/1
  Gain/1 -> Divide/1
  Chart/1(TxTrigger()) -> TxTrigger/1
  Divide/1 -> Data Type Conversion/1
  TxReq/1 -> Chart/1(TxReq)
  Constant/1 -> Divide/2
